simulink model "Seating"  (R2019a)
settings: Solver=FixedStepDiscrete  StartTime=0.0  StopTime=45  FixedStep=1  RelTol=1e-3
libraries: simulink x1
settings Model: Creator=admin  LastModifiedBy=admin
settings OptimizationCC: DefaultParameterBehavior=Inlined  EnhancedBackFolding=on  PassReuseOutputArgsAs=Individual arguments  OptimizeBlockOrder=speed  DifferentSizesBufferReuse=on  OptimizationCustomize=off
settings DebuggingCC: ParameterTunabilityLossMsg=error
settings SFSimCC: MATLABDynamicMemAlloc=off
settings RTWCC: SystemTargetFile=ert.tlc  TemplateMakefile=ert_default_tmf  GenerateReport=on  IncludeHyperlinkInReport=on  LaunchReport=on  GenerateTraceInfo=on  GenerateTraceReport=on  GenerateTraceReportSl=on  GenerateTraceReportSf=on  GenerateTraceReportEml=on
settings CodeAppCC: ForceParamTrailComments=on  IgnoreCustomStorageClasses=off  OperatorAnnotations=on  SimulinkDataObjDesc=on  SFDataObjDesc=on  InsertBlockDesc=on
settings ERTTargetCC: TargetLangStandard=C99 (ISO)  GenerateSampleERTMain=on  InlinedParameterPlacement=NonHierarchical  ERTCustomFileTemplate=example_file_process.tlc

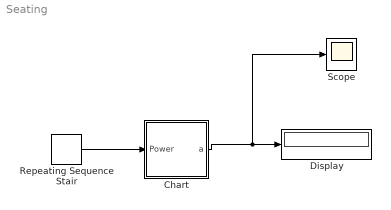
== system Seating ==
  Chart : Stateflow chart  BlockKeywords=__PRM__SERIALIZED__DATA__:Stateflow Chart,Stateflow Diagram  TreatAsAtomicUnit=on
  Display : Display
  Repeating Sequence Stair : simulink/Sources/Repeating Sequence Stair  OutValues=[1 1 1 1 1 0 1 1 1 1 0 1 1 1 10 1 0 1 1 0 1 ].'  tsamp=-1  OutMin=[]  OutMax=[]  OutDataTypeStr=double  OutputDataTypeScalingMode=double  OutDataType=fixdt(0,8)  ConRadixGroup=Best Precision: Vector-wise  OutScaling=2^-12
  Scope : Scope
  wires:
  Chart/1(a) -> Scope/1, Display/1
  Repeating Sequence Stair/1 -> Chart/1(Power)

== stateflow chart Seating/Chart ==
  state Power_ON_OFF
  state ON
    (history)
    state play_Stop
    state Run
      du:
      a=a
      (history)
      state forward
        en:a=0;
        du:a=a+5;
        ex:a=100;
      state backward
        en:a=100;
        du:a=a-5;
        ex:a=0;
      (default) -> forward
      forward -> backward : [a==100]
      backward -> forward : [a==0]
    (default) -> play_Stop
    play_Stop -> Run : [Power==1]
    Run -> play_Stop : [Power==0]
  (default) -> Power_ON_OFF
  Power_ON_OFF -> ON : [Power==1]
  ON -> Power_ON_OFF : [Power==0]
  data: a output; Power input
